simulink library "lib_resettable_unit_delay"  (R2023a)
settings: Solver=VariableStepAuto  StartTime=0.0  StopTime=10.0  RelTol=1e-3
settings Model: Creator=cav2ofo  LastModifiedBy=lenovo
settings OptimizationCC: ReuseModelBlockBuffer=off

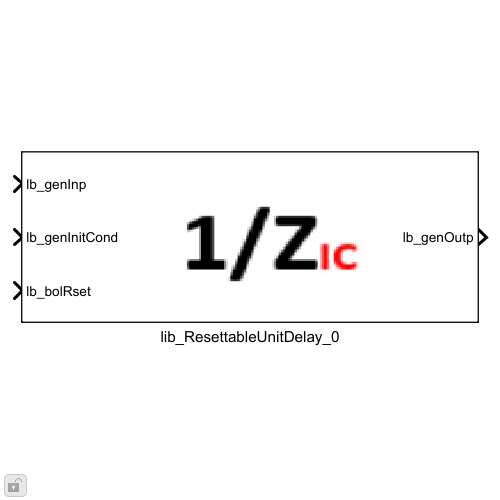
[thumbnail: Simulink's stored preview of the top-level diagram]
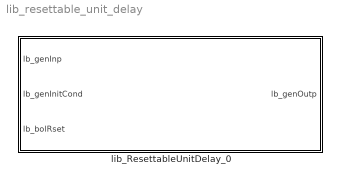
== system lib_resettable_unit_delay ==
  lib_ResettableUnitDelay_0 : Subsystem
      mask DialogControl DescGroupVar Prompt: VHIT control library
      mask DialogControl Control2 Prompt: Resettable unit delay
      mask Display: image('icons\resettable_unit_delay.png'); % Use "Edit Image" on toolstrip to change.

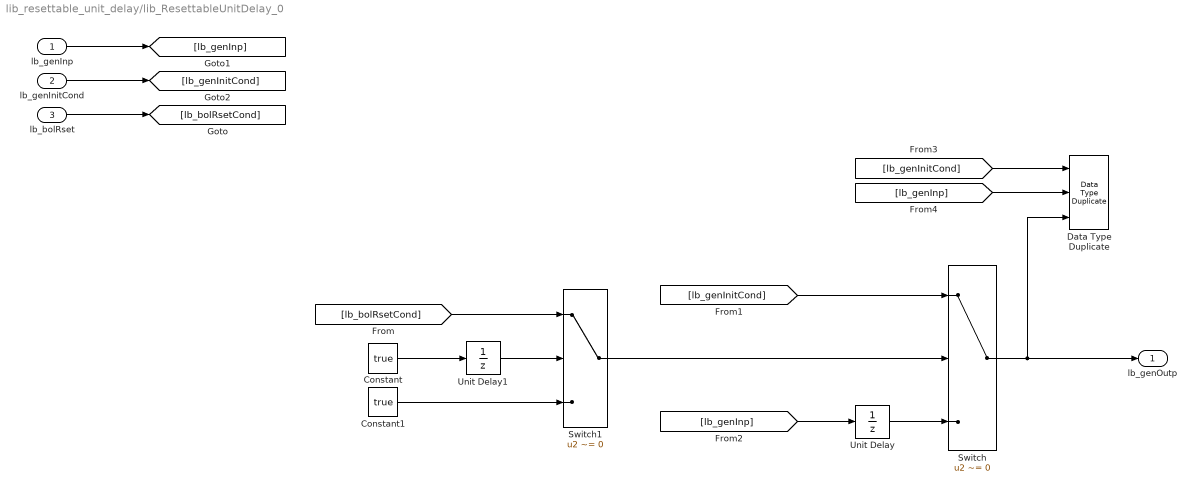
== system lib_resettable_unit_delay/lib_ResettableUnitDelay_0 ==
  lb_genInp : Inport
  lb_genInitCond : Inport  Port=2
  lb_bolRset : Inport  Port=3
  Constant : Constant  Value=true
  Constant1 : Constant  Value=true
  Data Type Duplicate : DataTypeDuplicate  NumInputPorts=3
  Switch : Switch  Criteria=u2 ~= 0  InputSameDT=off
  Switch1 : Switch  Criteria=u2 ~= 0  SaturateOnIntegerOverflow=off  InputSameDT=off
  Unit Delay : UnitDelay  SampleTime=-1  HasFrameUpgradeWarning=on
  Unit Delay1 : UnitDelay  InitialCondition=false  SampleTime=-1  HasFrameUpgradeWarning=on
  lb_genOutp : Outport  VectorParamsAs1DForOutWhenUnconnected=off
  wires:
  Unit Delay/1 -> Switch/3
  Switch/1 -> Data Type Duplicate/3, lb_genOutp/1
  Constant/1 -> Unit Delay1/1
  Unit Delay1/1 -> Switch1/2
  lb_bolRset/1 -> [lb_bolRsetCond]
  [lb_bolRsetCond] -> Switch1/1
  Constant1/1 -> Switch1/3
  Switch1/1 -> Switch/2
  lb_genInp/1 -> [lb_genInp]
  lb_genInitCond/1 -> [lb_genInitCond]
  [lb_genInp] -> Unit Delay/1
  [lb_genInitCond] -> Data Type Duplicate/1
  [lb_genInp] -> Data Type Duplicate/2
  [lb_genInitCond] -> Switch/1
